simulink model "Single_Use_Simulink_Switch"  (R2022b)
settings: Solver=FixedStepAuto  StartTime=0.0  StopTime=200  FixedStep=0.02  RelTol=1e-3
libraries: simulink x1
settings Model: Creator=Musta  LastModifiedBy=Musta

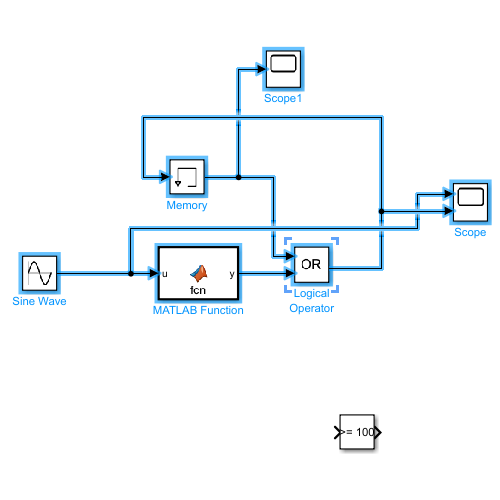
[thumbnail: Simulink's stored preview of the top-level diagram]
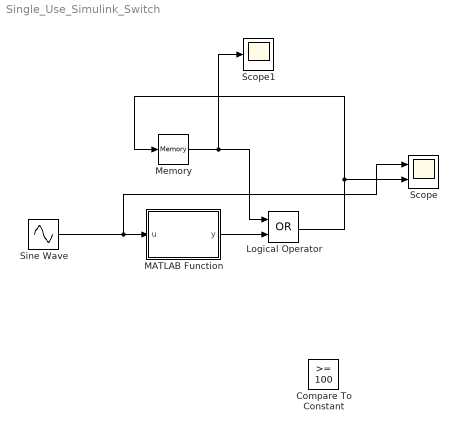
== system Single_Use_Simulink_Switch ==
  Compare To Constant : simulink/Logic and Bit Operations/Compare To Constant  relop=>=  const=100  OutDataTypeStr=boolean
  Logical Operator : Logic  Operator=OR  AllPortsSameDT=off  OutDataTypeStr=boolean
  MATLAB Function : MATLAB Function  TreatAsAtomicUnit=on
  Memory : Memory
  Scope : Scope  NumInputPorts=2
  Scope1 : Scope
  Sine Wave : Sin  Amplitude=200  Frequency=0.1  SampleTime=0
  wires:
  Sine Wave/1 -> MATLAB Function/1(u), Scope/1
  Logical Operator/1 -> Memory/1, Scope/2
  Memory/1 -> Scope1/1, Logical Operator/1
  MATLAB Function/1(y) -> Logical Operator/2

== matlab function Single_Use_Simulink_Switch/MATLAB Function ==
  data: u input; y output
function y = fcn(u)

    if u >= 100
        y = 1;
    else
        y = 0;
    end

end
